simulink model "Logic"  (Simulink 8.0)
settings: Solver=ode45  StartTime=0.0  StopTime=10.0  RelTol=1e-3
settings Model: Creator=Faradars  LastModifiedBy=Faradars

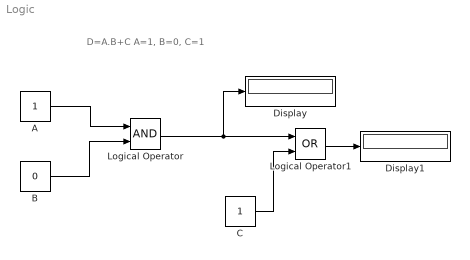
== system Logic ==
  note: D=A.B+C
      |
      | A=1, B=0, C=1
  A : Constant
  B : Constant  Value=0
  C : Constant
  Display : Display
  Display1 : Display
  Logical Operator : Logic  AllPortsSameDT=off  OutDataTypeStr=boolean
  Logical Operator1 : Logic  Operator=OR  AllPortsSameDT=off  OutDataTypeStr=boolean
  wires:
  A/1 -> Logical Operator/1
  B/1 -> Logical Operator/2
  C/1 -> Logical Operator1/2
  Logical Operator/1 -> Display/1, Logical Operator1/1
  Logical Operator1/1 -> Display1/1
